simulink model "linearInvPend_Pole_mdl"  (R2022b)
settings: Solver=ode4  StartTime=0.0  StopTime=0.5  FixedStep=.001  RelTol=1e-3
undefined symbols (not defined in the file): F, G, SS_0
settings Model: Creator=mo780715  LastModifiedBy=mohammadodeh

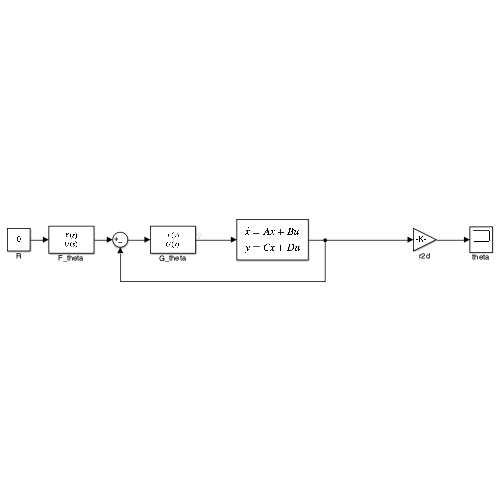
[thumbnail: Simulink's stored preview of the top-level diagram]
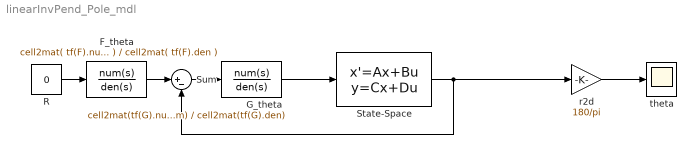
== system linearInvPend_Pole_mdl ==
  F_theta : TransferFcn  Numerator=cell2mat( tf(F).num )  Denominator=cell2mat( tf(F).den )
  G_theta : TransferFcn  Numerator=cell2mat(tf(G).num)  Denominator=cell2mat(tf(G).den)
  R : Constant  Value=0
  State-Space : StateSpace  A=SS_0.A  B=SS_0.B  C=SS_0.C  D=SS_0.D  InitialCondition=[ 0 5/180*pi /(-0.5) ]  ContinuousStateAttributes='theta'
  Sum : Sum  Inputs=|+-
  r2d : Gain  Gain=180/pi
  theta : Scope
  wires:
  r2d/1 -> theta/1
  State-Space/1 -> Sum/2, r2d/1
  G_theta/1 -> State-Space/1
  R/1 -> F_theta/1
  F_theta/1 -> Sum/1
  Sum/1 -> G_theta/1
